simulink model "CANConnectivityInAnAutomotiveApplication4"  (R2024a)
settings: Solver=VariableStepAuto  StartTime=0.0  StopTime=inf  RelTol=1e-3
model workspace (MAT data in the model file):
  k2 = 1e-06
undefined symbols (not defined in the file): canChannel, DiscIntNeverNeededParam
libraries: canmsglib x17, canlib x11, simulink x3
settings Model: Creator=The MathWorks, Inc.  LastModifiedBy=S D
settings SolverCC: AlgebraicLoopSolver=TrustRegion
settings DataIOCC: ReturnWorkspaceOutputs=off
settings DebuggingCC: UnconnectedInputMsg=warning  UnconnectedOutputMsg=warning  UnconnectedLineMsg=warning  ArithmeticOperatorsInVariantConditions=warning
settings ModelReferenceCC: EnableRefExpFcnMdlSchedulingChecks=on
settings SFSimCC: SimUseLocalCustomCode=off  CustomCodeUndefinedFunction=UseInterfaceOnly
settings RTWCC: RTWUseLocalCustomCode=off  GPUComputeCapability=3.5

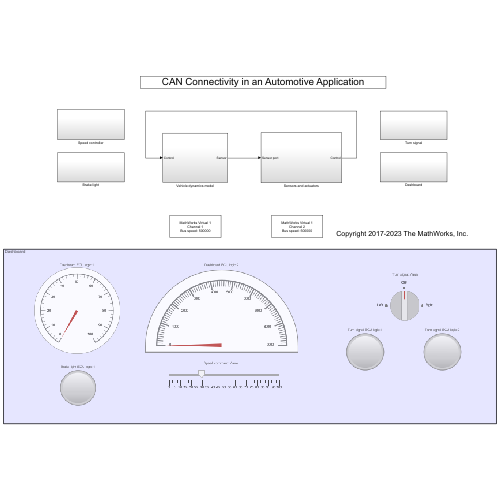
[thumbnail: Simulink's stored preview of the top-level diagram]
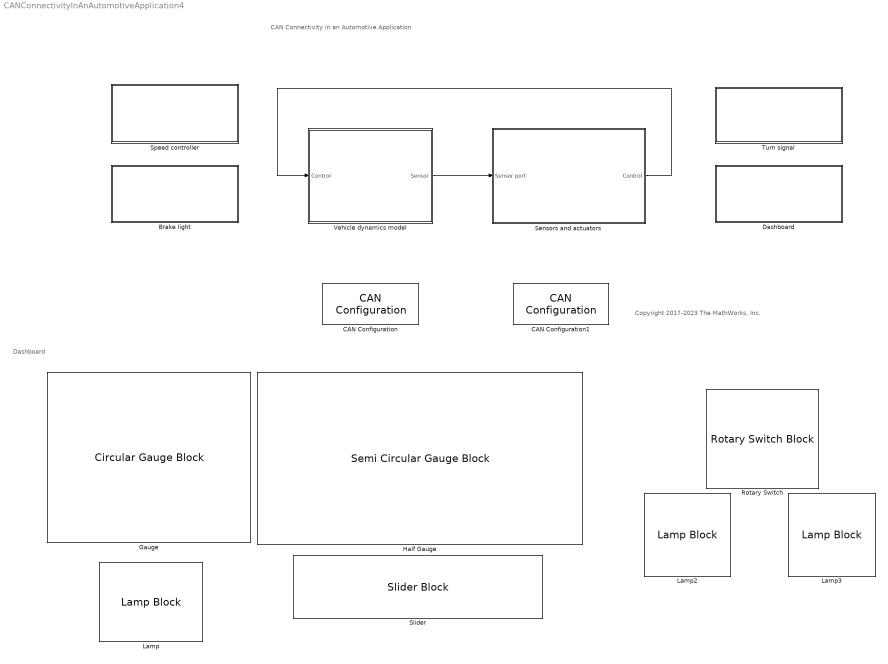
== system CANConnectivityInAnAutomotiveApplication4 ==
  note: Dashboard
  note: CAN Connectivity in an Automotive Application
  note: Copyright 2017-2023 The MathWorks, Inc.
  Brake light : Subsystem
  CAN Configuration : canlib/CAN Configuration  BlockHandle=1838.0012  Device=MathWorks Virtual 1 (Channel 1)  DeviceMenu=MathWorks Virtual 1 (Channel 1)  ObjConstructor=canChannel('MathWorks', 'Virtual 1', 1)  BusSpeed=500000  EnableBitParameters=off  AckMode=Normal
  CAN Configuration1 : canlib/CAN Configuration  BlockHandle=1839.0024  Device=MathWorks Virtual 1 (Channel 2)  DeviceMenu=MathWorks Virtual 1 (Channel 2)  ObjConstructor=canChannel('MathWorks', 'Virtual 1', 2)  BusSpeed=500000  EnableBitParameters=off  AckMode=Normal
  Dashboard : Subsystem
  Gauge : CircularGaugeBlock  TickInterval=10
  Half Gauge : SemiCircularGaugeBlock  ScaleMax=9000  TickInterval=1000
  Lamp : LampBlock
  Lamp2 : LampBlock
  Lamp3 : LampBlock
  Rotary Switch : RotarySwitchBlock
      settings: Values={{'Left', 'Off', 'Right'}, [1 2 3]}
  Sensors and actuators : Subsystem
  Slider : SliderBlock
  Speed controller : Subsystem
  Turn signal : Subsystem
  Vehicle dynamics model : Subsystem
  wires:
  Vehicle dynamics model/1(Sensor) -> Sensors and actuators/1(Sensor port)
  Sensors and actuators/1(Control) -> Vehicle dynamics model/1(Control)

== system CANConnectivityInAnAutomotiveApplication4/Brake light ==
  note: Brake light
  Brake light : Terminator
  Brake light ECU logic : Subsystem  TreatAsAtomicUnit=on
  CAN Receive : canlib/CAN Receive  BlockHandle=1831.002  Device=MathWorks Virtual 1 (Channel 2)  DeviceMenu=MathWorks Virtual 1 (Channel 2)  ObjConstructor=canChannel('MathWorks', 'Virtual 1', 2)  EnableStandardIDsFilter=off  StdIDsCombo=Allow all  StandardIDs=0  EnableExtendedIDsFilter=off  ExtIDsCombo=Allow all  ExtendedIDs=0  SampleTime=0.01  MsgsPerTimestep=all  InternalFilterUpdateStatus=on  BusOutput=on
  wires:
  CAN Receive/1 -> Brake light ECU logic/Trigger
  CAN Receive/2 -> Brake light ECU logic/1(CAN message)
  Brake light ECU logic/1(Brake status) -> Brake light/1

== system CANConnectivityInAnAutomotiveApplication4/Dashboard ==
  note: Dashboard
  CAN Receive : canlib/CAN Receive  BlockHandle=1841.0009  Device=MathWorks Virtual 1 (Channel 2)  DeviceMenu=MathWorks Virtual 1 (Channel 2)  ObjConstructor=canChannel('MathWorks', 'Virtual 1', 2)  EnableStandardIDsFilter=off  StdIDsCombo=Block all  StandardIDs=0  EnableExtendedIDsFilter=off  ExtIDsCombo=Allow all  ExtendedIDs=[50 100]  SampleTime=0.01  MsgsPerTimestep=all  InternalFilterUpdateStatus=on  BusOutput=on
  Dashboard ECU logic : Subsystem  TreatAsAtomicUnit=on
  Speedometer : Terminator
  Tachometer : Terminator
  wires:
  CAN Receive/1 -> Dashboard ECU logic/Trigger
  CAN Receive/2 -> Dashboard ECU logic/1(CAN message)
  Dashboard ECU logic/2(RPM) -> Tachometer/1
  Dashboard ECU logic/1(Speed) -> Speedometer/1

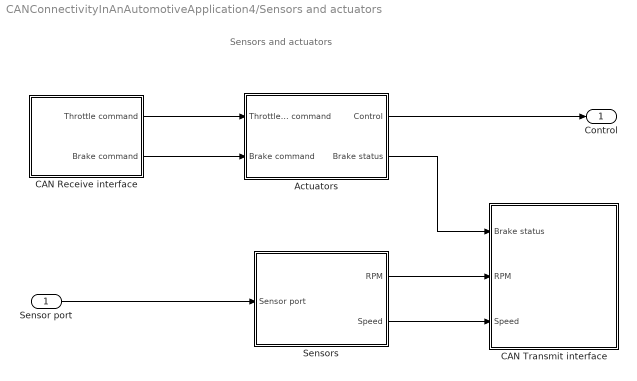
== system CANConnectivityInAnAutomotiveApplication4/Sensors and actuators ==
  note: Sensors and actuators
  Sensor port : Inport
  Actuators : Subsystem
  CAN Receive interface : Subsystem
  CAN Transmit interface : Subsystem
  Sensors : Subsystem
  Control : Outport  VectorParamsAs1DForOutWhenUnconnected=off
  wires:
  Sensor port/1 -> Sensors/1(Sensor port)
  Sensors/1(RPM) -> CAN Transmit interface/2(RPM)
  Sensors/2(Speed) -> CAN Transmit interface/3(Speed)
  Actuators/1(Control) -> Control/1
  Actuators/2(Brake status) -> CAN Transmit interface/1(Brake status)
  CAN Receive interface/1(Throttle command) -> Actuators/1(Throttle command)
  CAN Receive interface/2(Brake command) -> Actuators/2(Brake command)

== system CANConnectivityInAnAutomotiveApplication4/Speed controller ==
  note: Speed controller
  CAN Receive : canlib/CAN Receive  BlockHandle=2493.0005  Device=MathWorks Virtual 1 (Channel 2)  DeviceMenu=MathWorks Virtual 1 (Channel 2)  ObjConstructor=canChannel('MathWorks', 'Virtual 1', 2)  EnableStandardIDsFilter=off  StdIDsCombo=Allow all  StandardIDs=0  EnableExtendedIDsFilter=off  ExtIDsCombo=Allow all  ExtendedIDs=0  SampleTime=0.01  MsgsPerTimestep=all  InternalFilterUpdateStatus=on  BusOutput=on
  Speed controller ECU logic : Subsystem  TreatAsAtomicUnit=on
  wires:
  CAN Receive/1 -> Speed controller ECU logic/Trigger
  CAN Receive/2 -> Speed controller ECU logic/1(CAN message)

== system CANConnectivityInAnAutomotiveApplication4/Turn signal ==
  note: Turn signal
  CAN Receive : canlib/CAN Receive  BlockHandle=2632.0002  Device=MathWorks Virtual 1 (Channel 2)  DeviceMenu=MathWorks Virtual 1 (Channel 2)  ObjConstructor=canChannel('MathWorks', 'Virtual 1', 2)  EnableStandardIDsFilter=off  StdIDsCombo=Block all  StandardIDs=0  EnableExtendedIDsFilter=off  ExtIDsCombo=Allow all  ExtendedIDs=600  SampleTime=0.01  MsgsPerTimestep=all  InternalFilterUpdateStatus=on  BusOutput=on
  Left turn signal : Terminator
  Right turn signal : Terminator
  Turn signal ECU logic : Subsystem  TreatAsAtomicUnit=on
  wires:
  CAN Receive/1 -> Turn signal ECU logic/Trigger
  CAN Receive/2 -> Turn signal ECU logic/1(CAN message)
  Turn signal ECU logic/1(Left turn signal interface) -> Left turn signal/1
  Turn signal ECU logic/2(Right turn signal interface) -> Right turn signal/1

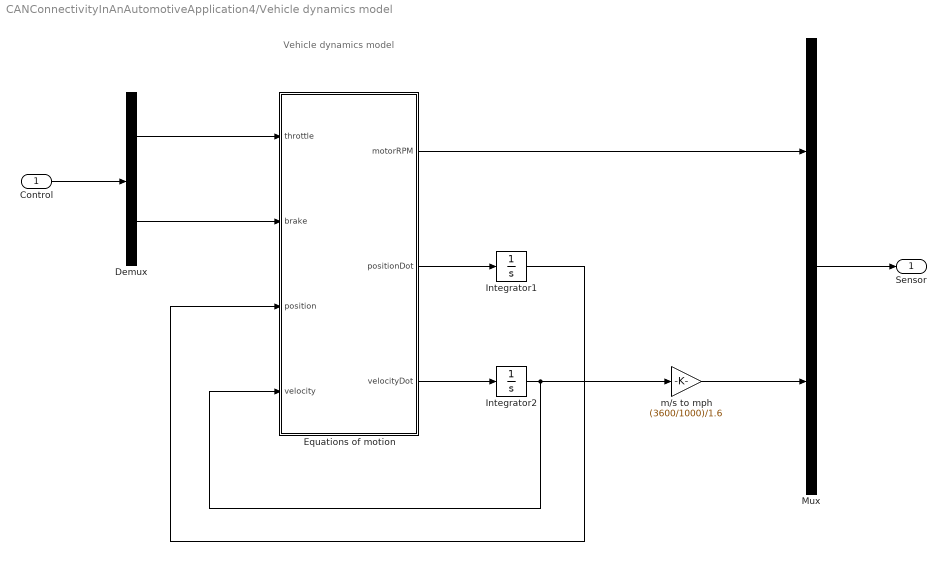
== system CANConnectivityInAnAutomotiveApplication4/Vehicle dynamics model ==
  note: Vehicle dynamics model
  Control : Inport
  Demux : Demux  Outputs=2
  Equations of motion : MATLAB Function  TreatAsAtomicUnit=on
  Integrator1 : Integrator
  Integrator2 : Integrator
  Mux : Mux  Inputs=2
  m/s to mph : Gain  Gain=(3600/1000)/1.6
  Sensor : Outport  VectorParamsAs1DForOutWhenUnconnected=off
  wires:
  Demux/1 -> Equations of motion/1(throttle)
  Equations of motion/2(positionDot) -> Integrator1/1
  Equations of motion/3(velocityDot) -> Integrator2/1
  Integrator2/1 -> m/s to mph/1, Equations of motion/4(velocity)
  Integrator1/1 -> Equations of motion/3(position)
  Demux/2 -> Equations of motion/2(brake)
  m/s to mph/1 -> Mux/2
  Equations of motion/1(motorRPM) -> Mux/1
  Control/1 -> Demux/1
  Mux/1 -> Sensor/1

== system CANConnectivityInAnAutomotiveApplication4/Brake light/Brake light ECU logic ==
  note: Brake light ECU logic
  CAN message : Inport
  function : TriggerPort  TriggerType=function-call  VariantControl=Variant
  CAN Unpack : canmsglib/CAN Unpack  CANdbFile=canConnectivityForVehicle.dbc  MsgList=BrakeStatusMessage  MsgName=BrakeStatusMessage  MsgIDType=Extended (29-bit identifier)  MsgIdentifier=1280  MsgLength=1  SignalInfo={'BrakeStatus','0','1','LE','unsigned','Standard','0','1','0','0','1'}  IDPort=off  TimestampPort=off  ErrorPort=off  RemotePort=off  LengthPort=off  StatusPort=off  ApplyMinMax=off
      settings: DataFormat=CANdb specified signals
  Brake status : Outport  VectorParamsAs1DForOutWhenUnconnected=off
  wires:
  CAN message/1 -> CAN Unpack/1
  CAN Unpack/1 -> Brake status/1

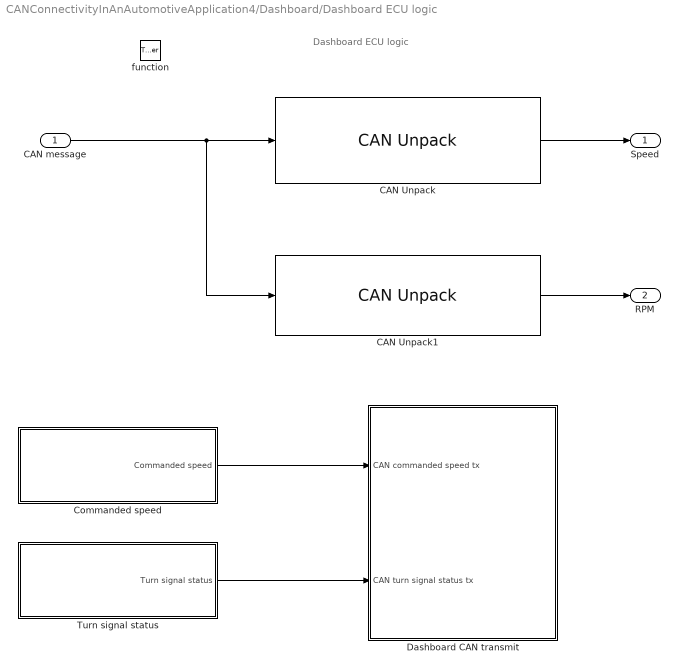
== system CANConnectivityInAnAutomotiveApplication4/Dashboard/Dashboard ECU logic ==
  note: Dashboard ECU logic
  CAN message : Inport
  function : TriggerPort  TriggerType=function-call  VariantControl=Variant
  CAN Unpack : canmsglib/CAN Unpack  CANdbFile=canConnectivityForVehicle.dbc  MsgList=SpeedMessage  MsgName=SpeedMessage  MsgIDType=Extended (29-bit identifier)  MsgIdentifier=256  MsgLength=8  SignalInfo={'Speed','0','64','LE','double','Standard','0','1','0','0','100'}  IDPort=off  TimestampPort=off  ErrorPort=off  RemotePort=off  LengthPort=off  StatusPort=off  ApplyMinMax=off
      settings: DataFormat=CANdb specified signals
  CAN Unpack1 : canmsglib/CAN Unpack  CANdbFile=canConnectivityForVehicle.dbc  MsgList=RPMMessage  MsgName=RPMMessage  MsgIDType=Extended (29-bit identifier)  MsgIdentifier=2048  MsgLength=8  SignalInfo={'RPM','0','64','LE','double','Standard','0','1','0','0','10000'}  IDPort=off  TimestampPort=off  ErrorPort=off  RemotePort=off  LengthPort=off  StatusPort=off  ApplyMinMax=off
      settings: DataFormat=CANdb specified signals
  Commanded speed : Subsystem
  Dashboard CAN transmit : Subsystem
  Turn signal status : Subsystem
  Speed : Outport  VectorParamsAs1DForOutWhenUnconnected=off
  RPM : Outport  Port=2  VectorParamsAs1DForOutWhenUnconnected=off
  wires:
  CAN message/1 -> CAN Unpack1/1, CAN Unpack/1
  Turn signal status/1(Turn signal status) -> Dashboard CAN transmit/2(CAN turn signal status tx)
  Commanded speed/1(Commanded speed) -> Dashboard CAN transmit/1(CAN commanded speed tx)
  CAN Unpack/1 -> Speed/1
  CAN Unpack1/1 -> RPM/1

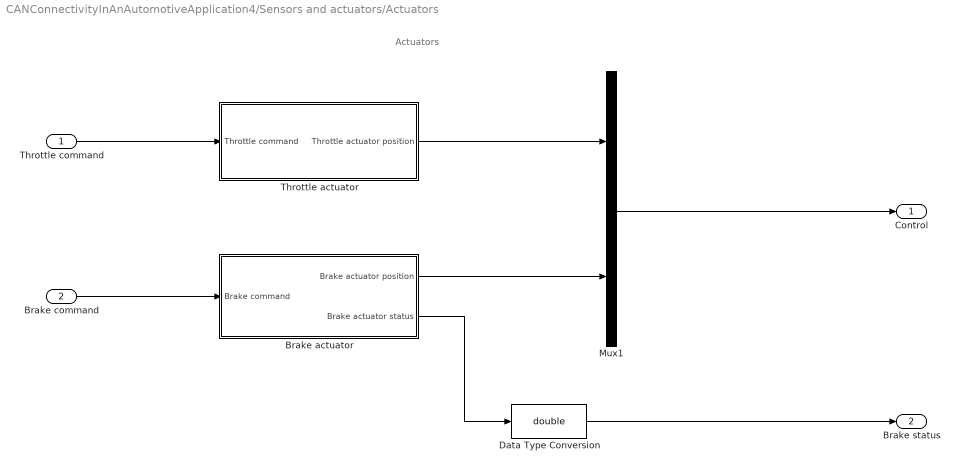
== system CANConnectivityInAnAutomotiveApplication4/Sensors and actuators/Actuators ==
  note: Actuators
  Throttle command : Inport
  Brake command : Inport  Port=2
  Brake actuator : Subsystem
  Data Type Conversion : DataTypeConversion  OutDataTypeStr=double  SaturateOnIntegerOverflow=off  RndMeth=Floor
  Mux1 : Mux  Inputs=2
  Throttle actuator : Subsystem
  Control : Outport  VectorParamsAs1DForOutWhenUnconnected=off
  Brake status : Outport  Port=2  VectorParamsAs1DForOutWhenUnconnected=off
  wires:
  Brake actuator/1(Brake actuator position) -> Mux1/2
  Throttle actuator/1(Throttle actuator position) -> Mux1/1
  Brake command/1 -> Brake actuator/1(Brake command)
  Throttle command/1 -> Throttle actuator/1(Throttle command)
  Data Type Conversion/1 -> Brake status/1
  Brake actuator/2(Brake actuator status) -> Data Type Conversion/1
  Mux1/1 -> Control/1

== system CANConnectivityInAnAutomotiveApplication4/Sensors and actuators/CAN Receive interface ==
  note: CAN Receive interface
  CAN Receive : canlib/CAN Receive  BlockHandle=2311.0005  Device=MathWorks Virtual 1 (Channel 1)  DeviceMenu=MathWorks Virtual 1 (Channel 1)  ObjConstructor=canChannel('MathWorks', 'Virtual 1', 1)  EnableStandardIDsFilter=off  StdIDsCombo=Allow all  StandardIDs=0  EnableExtendedIDsFilter=off  ExtIDsCombo=Allow all  ExtendedIDs=0  SampleTime=0.01  MsgsPerTimestep=all  InternalFilterUpdateStatus=off  BusOutput=on
  Extract message : Subsystem  TreatAsAtomicUnit=on
  Throttle command : Outport  VectorParamsAs1DForOutWhenUnconnected=off
  Brake command : Outport  Port=2  VectorParamsAs1DForOutWhenUnconnected=off
  wires:
  CAN Receive/1 -> Extract message/Trigger
  CAN Receive/2 -> Extract message/1(In1)
  Extract message/1(Throttle command) -> Throttle command/1
  Extract message/2(Brake actuator position) -> Brake command/1

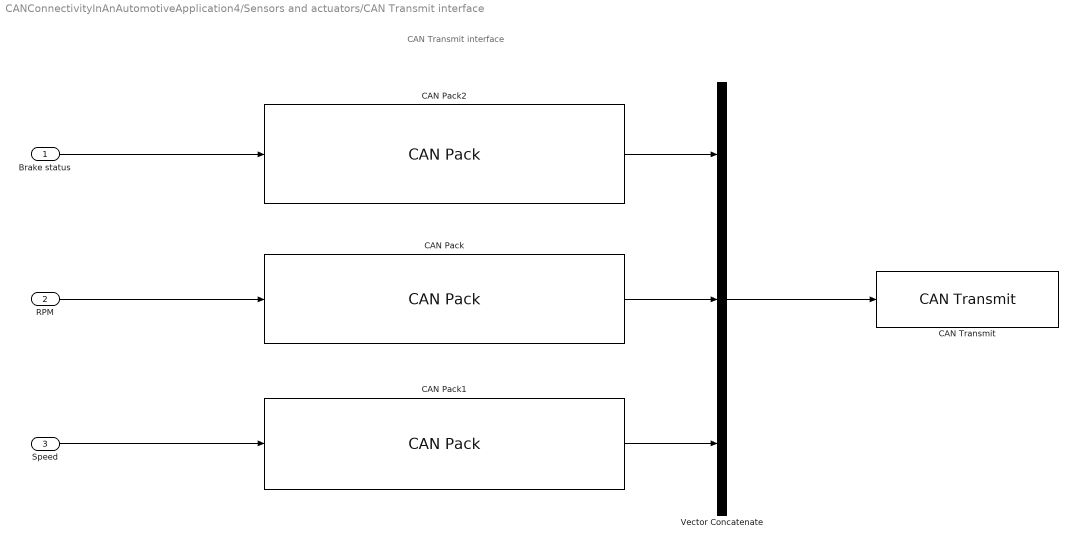
== system CANConnectivityInAnAutomotiveApplication4/Sensors and actuators/CAN Transmit interface ==
  note: CAN Transmit interface
  Brake status : Inport
  RPM : Inport  Port=2
  Speed : Inport  Port=3
  CAN Pack : canmsglib/CAN Pack  CANdbFile=canConnectivityForVehicle.dbc  MsgList=RPMMessage  MsgName=RPMMessage  MsgIDType=Extended (29-bit identifier)  MsgIdentifier=2048  MsgLength=8  Remote=off  ApplyMinMax=off  BusOutput=on  SignalInfo={'RPM','0','64','LE','double','Standard','0','1','0','0','10000'}
      settings: DataFormat=CANdb specified signals
  CAN Pack1 : canmsglib/CAN Pack  CANdbFile=canConnectivityForVehicle.dbc  MsgList=SpeedMessage  MsgName=SpeedMessage  MsgIDType=Extended (29-bit identifier)  MsgIdentifier=256  MsgLength=8  Remote=off  ApplyMinMax=off  BusOutput=on  SignalInfo={'Speed','0','64','LE','double','Standard','0','1','0','0','100'}
      settings: DataFormat=CANdb specified signals
  CAN Pack2 : canmsglib/CAN Pack  CANdbFile=canConnectivityForVehicle.dbc  MsgList=BrakeStatusMessage  MsgName=BrakeStatusMessage  MsgIDType=Extended (29-bit identifier)  MsgIdentifier=1280  MsgLength=1  Remote=off  ApplyMinMax=off  BusOutput=on  SignalInfo={'BrakeStatus','0','1','LE','unsigned','Standard','0','1','0','0','1'}
      settings: DataFormat=CANdb specified signals
  CAN Transmit : canlib/CAN Transmit  BlockHandle=2420.0005  Device=MathWorks Virtual 1 (Channel 1)  DeviceMenu=MathWorks Virtual 1 (Channel 1)  ObjConstructor=canChannel('MathWorks', 'Virtual 1', 1)  EnableEventTransmit=off  EnablePeriodicTransmit=off  MessagePeriod=1.000
  Vector Concatenate : Concatenate  NumInputs=3
  wires:
  Speed/1 -> CAN Pack1/1
  Brake status/1 -> CAN Pack2/1
  CAN Pack1/1 -> Vector Concatenate/3
  Vector Concatenate/1 -> CAN Transmit/1
  CAN Pack/1 -> Vector Concatenate/2
  CAN Pack2/1 -> Vector Concatenate/1
  RPM/1 -> CAN Pack/1

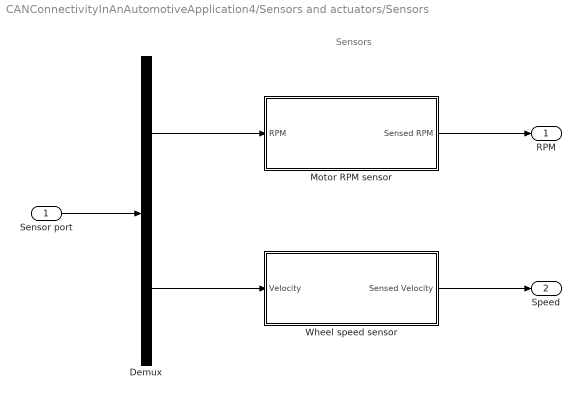
== system CANConnectivityInAnAutomotiveApplication4/Sensors and actuators/Sensors ==
  note: Sensors
  Sensor port : Inport
  Demux : Demux  Outputs=2
  Motor RPM sensor : Subsystem
  Wheel speed sensor : Subsystem
  RPM : Outport  VectorParamsAs1DForOutWhenUnconnected=off
  Speed : Outport  Port=2  VectorParamsAs1DForOutWhenUnconnected=off
  wires:
  Motor RPM sensor/1(Sensed RPM) -> RPM/1
  Wheel speed sensor/1(Sensed Velocity) -> Speed/1
  Demux/1 -> Motor RPM sensor/1(RPM)
  Demux/2 -> Wheel speed sensor/1(Velocity)
  Sensor port/1 -> Demux/1

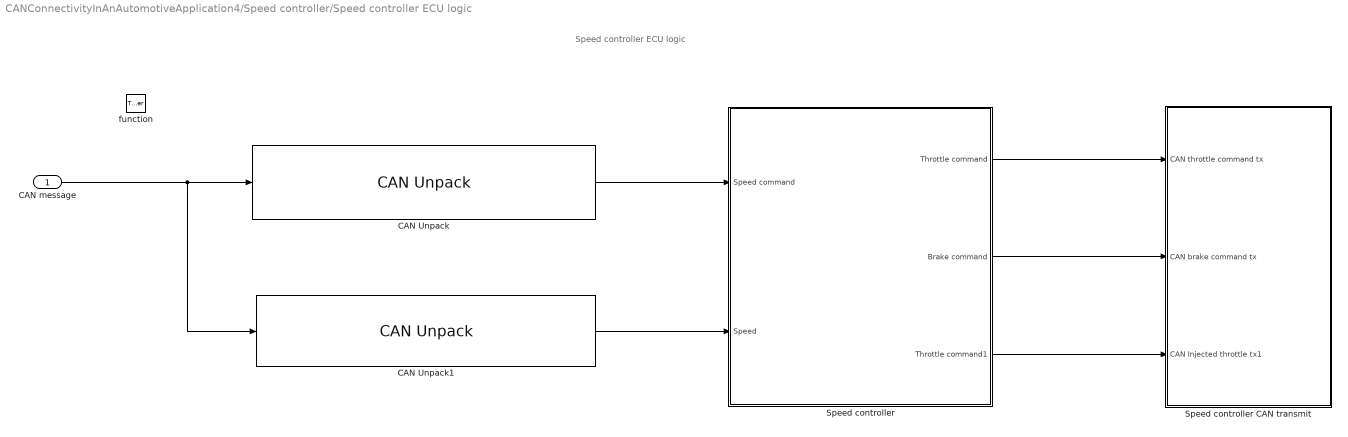
== system CANConnectivityInAnAutomotiveApplication4/Speed controller/Speed controller ECU logic ==
  note: Speed controller ECU logic
  CAN message : Inport
  function : TriggerPort  TriggerType=function-call  VariantControl=Variant
  CAN Unpack : canmsglib/CAN Unpack  CANdbFile=canConnectivityForVehicle.dbc  MsgList=SpeedCommandMessage  MsgName=SpeedCommandMessage  MsgIDType=Extended (29-bit identifier)  MsgIdentifier=1024  MsgLength=8  SignalInfo={'SpeedCommand','0','64','LE','double','Standard','0','1','0','0','100'}  IDPort=off  TimestampPort=off  ErrorPort=off  RemotePort=off  LengthPort=off  StatusPort=off  ApplyMinMax=off
      settings: DataFormat=CANdb specified signals
  CAN Unpack1 : canmsglib/CAN Unpack  CANdbFile=canConnectivityForVehicle.dbc  MsgList=SpeedMessage  MsgName=SpeedMessage  MsgIDType=Extended (29-bit identifier)  MsgIdentifier=256  MsgLength=8  SignalInfo={'Speed','0','64','LE','double','Standard','0','1','0','0','100'}  IDPort=off  TimestampPort=off  ErrorPort=off  RemotePort=off  LengthPort=off  StatusPort=off  ApplyMinMax=off
      settings: DataFormat=CANdb specified signals
  Speed controller : Subsystem
  Speed controller CAN transmit : Subsystem
  wires:
  CAN message/1 -> CAN Unpack1/1, CAN Unpack/1
  Speed controller/1(Throttle command) -> Speed controller CAN transmit/1(CAN throttle command tx)
  Speed controller/2(Brake command) -> Speed controller CAN transmit/2(CAN brake command tx)
  CAN Unpack/1 -> Speed controller/1(Speed command)
  CAN Unpack1/1 -> Speed controller/2(Speed)
  Speed controller/3(Throttle command1) -> Speed controller CAN transmit/3(CAN Injected throttle tx1)

== system CANConnectivityInAnAutomotiveApplication4/Turn signal/Turn signal ECU logic ==
  note: Turn signal ECU logic
  CAN message : Inport
  function : TriggerPort  TriggerType=function-call  VariantControl=Variant
  CAN Unpack : canmsglib/CAN Unpack  CANdbFile=canConnectivityForVehicle.dbc  MsgList=TurnSignalStatusMessage  MsgName=TurnSignalStatusMessage  MsgIDType=Extended (29-bit identifier)  MsgIdentifier=1536  MsgLength=1  SignalInfo={'TurnSignalStatus','0','3','LE','unsigned','Standard','0','1','0','1','3'}  IDPort=off  TimestampPort=off  ErrorPort=off  RemotePort=off  LengthPort=off  StatusPort=off  ApplyMinMax=off
      settings: DataFormat=CANdb specified signals
  Turn signal logic : Subsystem
  Left turn signal interface : Outport  VectorParamsAs1DForOutWhenUnconnected=off
  Right turn signal interface : Outport  Port=2  VectorParamsAs1DForOutWhenUnconnected=off
  wires:
  CAN message/1 -> CAN Unpack/1
  CAN Unpack/1 -> Turn signal logic/1(Turn signal status)
  Turn signal logic/1(Left turn signal interface) -> Left turn signal interface/1
  Turn signal logic/2(Right turn signal interface) -> Right turn signal interface/1

== system CANConnectivityInAnAutomotiveApplication4/Dashboard/Dashboard ECU logic/Commanded speed ==
  note: Commanded speed
  Speed command : Constant  Value=42.53198205682007  OutDataTypeStr=double  SampleTime=Inf
  Zero-Order Hold : ZeroOrderHold  SampleTime=-1
  Commanded speed : Outport  VectorParamsAs1DForOutWhenUnconnected=off
  wires:
  Speed command/1 -> Zero-Order Hold/1
  Zero-Order Hold/1 -> Commanded speed/1

== system CANConnectivityInAnAutomotiveApplication4/Dashboard/Dashboard ECU logic/Dashboard CAN transmit ==
  note: Dashboard CAN transmit
  CAN commanded speed tx : Inport
  CAN turn signal status tx : Inport  Port=2
  CAN Pack : canmsglib/CAN Pack  CANdbFile=canConnectivityForVehicle.dbc  MsgList=TurnSignalStatusMessage  MsgName=TurnSignalStatusMessage  MsgIDType=Extended (29-bit identifier)  MsgIdentifier=1536  MsgLength=1  Remote=off  ApplyMinMax=off  BusOutput=on  SignalInfo={'TurnSignalStatus','0','3','LE','unsigned','Standard','0','1','0','1','3'}
      settings: DataFormat=CANdb specified signals
  CAN Pack1 : canmsglib/CAN Pack  CANdbFile=canConnectivityForVehicle.dbc  MsgList=SpeedCommandMessage  MsgName=SpeedCommandMessage  MsgIDType=Extended (29-bit identifier)  MsgIdentifier=1024  MsgLength=8  Remote=off  ApplyMinMax=off  BusOutput=on  SignalInfo={'SpeedCommand','0','64','LE','double','Standard','0','1','0','0','100'}
      settings: DataFormat=CANdb specified signals
  CAN Transmit : canlib/CAN Transmit  BlockHandle=1905.0026  Device=MathWorks Virtual 1 (Channel 1)  DeviceMenu=MathWorks Virtual 1 (Channel 1)  ObjConstructor=canChannel('MathWorks', 'Virtual 1', 1)  EnableEventTransmit=off  EnablePeriodicTransmit=on  MessagePeriod=0.01
  CAN Transmit1 : canlib/CAN Transmit  BlockHandle=1907.0023  Device=MathWorks Virtual 1 (Channel 1)  DeviceMenu=MathWorks Virtual 1 (Channel 1)  ObjConstructor=canChannel('MathWorks', 'Virtual 1', 1)  EnableEventTransmit=off  EnablePeriodicTransmit=on  MessagePeriod=0.01
  wires:
  CAN commanded speed tx/1 -> CAN Pack1/1
  CAN Pack/1 -> CAN Transmit/1
  CAN turn signal status tx/1 -> CAN Pack/1
  CAN Pack1/1 -> CAN Transmit1/1

== system CANConnectivityInAnAutomotiveApplication4/Dashboard/Dashboard ECU logic/Turn signal status ==
  note: Turn signal status
  Turn signal : Constant  Value=2  OutDataTypeStr=double
  Zero-Order Hold : ZeroOrderHold  SampleTime=-1
  Turn signal status : Outport  VectorParamsAs1DForOutWhenUnconnected=off
  wires:
  Turn signal/1 -> Zero-Order Hold/1
  Zero-Order Hold/1 -> Turn signal status/1

== system CANConnectivityInAnAutomotiveApplication4/Sensors and actuators/Actuators/Brake actuator ==
  note: Brake actuator
  Brake command : Inport
  Brake actuator : TransferFcn  Denominator=[0.1 1]
  Brake status sensor : Subsystem
  Brake actuator position : Outport  VectorParamsAs1DForOutWhenUnconnected=off
  Brake actuator status : Outport  Port=2  VectorParamsAs1DForOutWhenUnconnected=off
  wires:
  Brake status sensor/1(Brake status) -> Brake actuator status/1
  Brake command/1 -> Brake actuator/1
  Brake actuator/1 -> Brake actuator position/1, Brake status sensor/1(Brake actuator position)

== system CANConnectivityInAnAutomotiveApplication4/Sensors and actuators/Actuators/Throttle actuator ==
  note: Throttle actuator
  Throttle command : Inport
  Throttle actuator : TransferFcn  Denominator=[0.1 1]
  Throttle actuator position : Outport  VectorParamsAs1DForOutWhenUnconnected=off
  wires:
  Throttle command/1 -> Throttle actuator/1
  Throttle actuator/1 -> Throttle actuator position/1

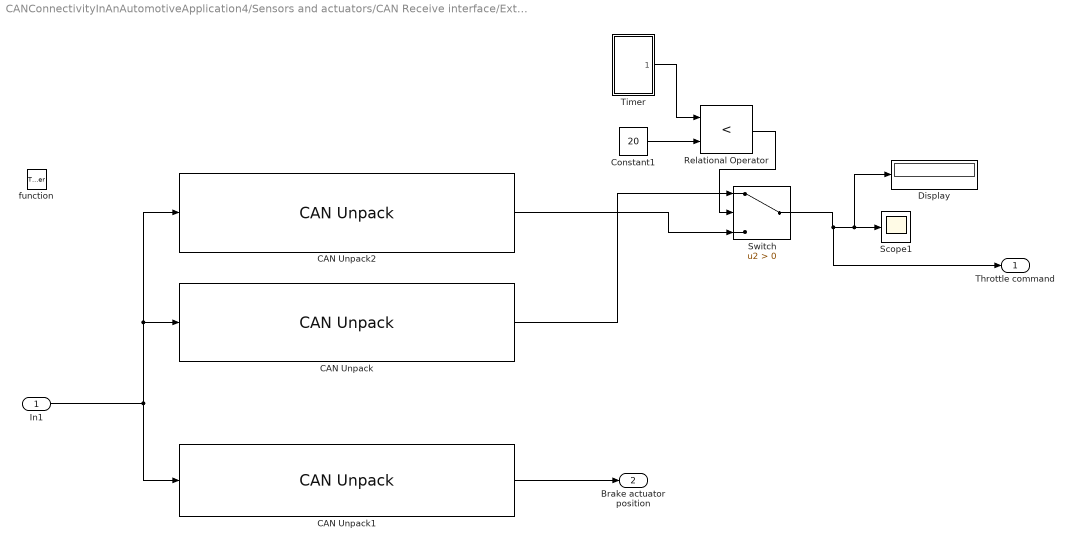
== system CANConnectivityInAnAutomotiveApplication4/Sensors and actuators/CAN Receive interface/Extract message ==
  In1 : Inport
  function : TriggerPort  TriggerType=function-call  VariantControl=Variant
  CAN Unpack : canmsglib/CAN Unpack  CANdbFile=canConnectivityForVehicle.dbc  MsgList=ThrottleCommandMessage  MsgName=ThrottleCommandMessage  MsgIDType=Extended (29-bit identifier)  MsgIdentifier=96  MsgLength=8  SignalInfo={'ThrottleCommand','0','64','LE','double','Standard','0','1','0','0','1'}  IDPort=off  TimestampPort=off  ErrorPort=off  RemotePort=off  LengthPort=off  StatusPort=off  ApplyMinMax=off
      settings: DataFormat=CANdb specified signals
  CAN Unpack1 : canmsglib/CAN Unpack  CANdbFile=canConnectivityForVehicle.dbc  MsgList=BrakeCommandMessage  MsgName=BrakeCommandMessage  MsgIDType=Extended (29-bit identifier)  MsgIdentifier=81  MsgLength=8  SignalInfo={'BrakeCommand','0','64','LE','double','Standard','0','1','0','0','1'}  IDPort=off  TimestampPort=off  ErrorPort=off  RemotePort=off  LengthPort=off  StatusPort=off  ApplyMinMax=off
      settings: DataFormat=CANdb specified signals
  CAN Unpack2 : canmsglib/CAN Unpack  CANdbFile=canConnectivityForVehicle.dbc  MsgList=InjectedThrottleMessage  MsgName=InjectedThrottleMessage  MsgIDType=Extended (29-bit identifier)  MsgIdentifier=95  MsgLength=8  SignalInfo={'InjectedThrottle','0','64','LE','double','Standard','0','0.5','0','0','0.5'}  IDPort=off  TimestampPort=off  ErrorPort=off  RemotePort=off  LengthPort=off  StatusPort=off  ApplyMinMax=off
      settings: DataFormat=CANdb specified signals
  Constant1 : Constant  Value=20
  Display : Display
  Relational Operator : RelationalOperator  Operator=<  OutDataTypeStr=boolean  RndMeth=Simplest  InputSameDT=off
  Scope1 : Scope
  Switch : Switch  Criteria=u2 > Threshold  SaturateOnIntegerOverflow=off  InputSameDT=off
  Timer : Subsystem
  Throttle command : Outport  VectorParamsAs1DForOutWhenUnconnected=off
  Brake actuator position : Outport  Port=2  VectorParamsAs1DForOutWhenUnconnected=off
  wires:
  In1/1 -> CAN Unpack1/1, CAN Unpack2/1, CAN Unpack/1
  CAN Unpack1/1 -> Brake actuator position/1
  Relational Operator/1 -> Switch/2
  Timer/1(Outport) -> Relational Operator/1
  Constant1/1 -> Relational Operator/2
  Switch/1 -> Throttle command/1, Display/1, Scope1/1
  CAN Unpack/1 -> Switch/1
  CAN Unpack2/1 -> Switch/3

== system CANConnectivityInAnAutomotiveApplication4/Sensors and actuators/Sensors/Motor RPM sensor ==
  note: Motor RPM sensor
  RPM : Inport
  Zero-Order Hold : ZeroOrderHold  SampleTime=.01
  Sensed RPM : Outport  VectorParamsAs1DForOutWhenUnconnected=off
  wires:
  Zero-Order Hold/1 -> Sensed RPM/1
  RPM/1 -> Zero-Order Hold/1

== system CANConnectivityInAnAutomotiveApplication4/Sensors and actuators/Sensors/Wheel speed sensor ==
  note: Wheel speed sensor
  Velocity : Inport
  Zero-Order Hold : ZeroOrderHold  SampleTime=.01
  Sensed Velocity : Outport  VectorParamsAs1DForOutWhenUnconnected=off
  wires:
  Zero-Order Hold/1 -> Sensed Velocity/1
  Velocity/1 -> Zero-Order Hold/1

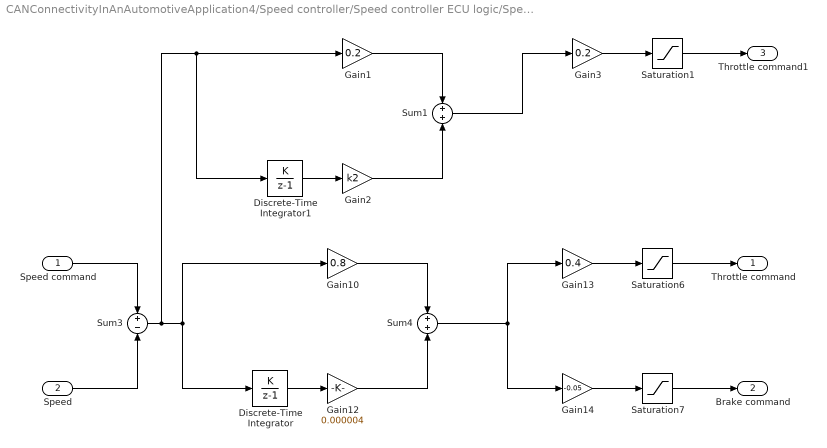
== system CANConnectivityInAnAutomotiveApplication4/Speed controller/Speed controller ECU logic/Speed controller ==
  Speed command : Inport
  Speed : Inport  Port=2
  Discrete-Time Integrator : DiscreteIntegrator  IntegratorMethod=Accumulation: Forward Euler  SampleTime=-1  ICPrevOutput=DiscIntNeverNeededParam  ICPrevScaledInput=DiscIntNeverNeededParam
  Discrete-Time Integrator1 : DiscreteIntegrator  IntegratorMethod=Accumulation: Forward Euler  SampleTime=-1  ICPrevOutput=DiscIntNeverNeededParam  ICPrevScaledInput=DiscIntNeverNeededParam
  Gain1 : Gain  Gain=0.2
  Gain10 : Gain  Gain=0.8
  Gain12 : Gain  Gain=0.000004
  Gain13 : Gain  Gain=0.4
  Gain14 : Gain  Gain=-0.05
  Gain2 : Gain  Gain=k2
  Gain3 : Gain  Gain=0.2
  Saturation1 : Saturate  UpperLimit=1  LowerLimit=0
  Saturation6 : Saturate  UpperLimit=1  LowerLimit=0
  Saturation7 : Saturate  UpperLimit=1  LowerLimit=0
  Sum1 : Sum  Inputs=+|+
  Sum3 : Sum  Inputs=+|-
  Sum4 : Sum  Inputs=+|+
  Throttle command : Outport  VectorParamsAs1DForOutWhenUnconnected=off
  Brake command : Outport  Port=2  VectorParamsAs1DForOutWhenUnconnected=off
  Throttle command1 : Outport  Port=3  VectorParamsAs1DForOutWhenUnconnected=off
  wires:
  Saturation7/1 -> Brake command/1
  Saturation6/1 -> Throttle command/1
  Speed command/1 -> Sum3/1
  Speed/1 -> Sum3/2
  Sum3/1 -> Discrete-Time Integrator1/1, Gain1/1, Discrete-Time Integrator/1, Gain10/1
  Discrete-Time Integrator/1 -> Gain12/1
  Gain10/1 -> Sum4/1
  Sum4/1 -> Gain14/1, Gain13/1
  Gain14/1 -> Saturation7/1
  Gain13/1 -> Saturation6/1
  Gain12/1 -> Sum4/2
  Gain3/1 -> Saturation1/1
  Saturation1/1 -> Throttle command1/1
  Gain2/1 -> Sum1/2
  Gain1/1 -> Sum1/1
  Discrete-Time Integrator1/1 -> Gain2/1
  Sum1/1 -> Gain3/1

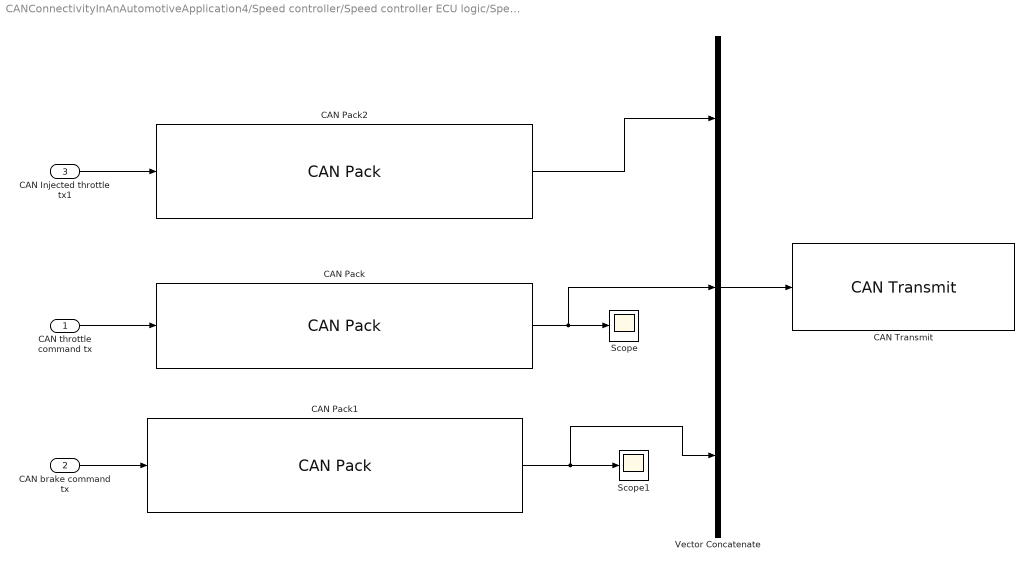
== system CANConnectivityInAnAutomotiveApplication4/Speed controller/Speed controller ECU logic/Speed controller CAN transmit ==
  CAN throttle command tx : Inport
  CAN brake command tx : Inport  Port=2
  CAN Injected throttle tx1 : Inport  Port=3
  CAN Pack : canmsglib/CAN Pack  CANdbFile=canConnectivityForVehicle.dbc  MsgList=ThrottleCommandMessage  MsgName=ThrottleCommandMessage  MsgIDType=Extended (29-bit identifier)  MsgIdentifier=96  MsgLength=8  Remote=off  ApplyMinMax=off  BusOutput=on  SignalInfo={'ThrottleCommand','0','64','LE','double','Standard','0','1','0','0','1'}
      settings: DataFormat=CANdb specified signals
  CAN Pack1 : canmsglib/CAN Pack  CANdbFile=canConnectivityForVehicle.dbc  MsgList=BrakeCommandMessage  MsgName=BrakeCommandMessage  MsgIDType=Extended (29-bit identifier)  MsgIdentifier=81  MsgLength=8  Remote=off  ApplyMinMax=off  BusOutput=on  SignalInfo={'BrakeCommand','0','64','LE','double','Standard','0','1','0','0','1'}
      settings: DataFormat=CANdb specified signals
  CAN Pack2 : canmsglib/CAN Pack  CANdbFile=canConnectivityForVehicle.dbc  MsgList=InjectedThrottleMessage  MsgName=InjectedThrottleMessage  MsgIDType=Extended (29-bit identifier)  MsgIdentifier=95  MsgLength=8  Remote=off  ApplyMinMax=off  BusOutput=on  SignalInfo={'InjectedThrottle','0','64','LE','double','Standard','0','0.5','0','0','0.5'}
      settings: DataFormat=CANdb specified signals
  CAN Transmit : canlib/CAN Transmit  BlockHandle=2597.0002  Device=MathWorks Virtual 1 (Channel 1)  DeviceMenu=MathWorks Virtual 1 (Channel 1)  ObjConstructor=canChannel('MathWorks', 'Virtual 1', 1)  EnableEventTransmit=off  EnablePeriodicTransmit=on  MessagePeriod=0.01
  Scope : Scope
  Scope1 : Scope
  Vector Concatenate : Concatenate  NumInputs=3
  wires:
  CAN Pack/1 -> Vector Concatenate/2, Scope/1
  CAN throttle command tx/1 -> CAN Pack/1
  CAN brake command tx/1 -> CAN Pack1/1
  Vector Concatenate/1 -> CAN Transmit/1
  CAN Pack1/1 -> Vector Concatenate/3, Scope1/1
  CAN Injected throttle tx1/1 -> CAN Pack2/1
  CAN Pack2/1 -> Vector Concatenate/1

== system CANConnectivityInAnAutomotiveApplication4/Turn signal/Turn signal ECU logic/Turn signal logic ==
  note: Turn signal logic
  Turn signal status : Inport
  Compare To Constant1 : simulink/Logic and Bit Operations/Compare To Constant  relop===  const=1  OutDataTypeStr=boolean
  Compare To Constant2 : simulink/Logic and Bit Operations/Compare To Constant  relop===  const=3  OutDataTypeStr=boolean
  Left turn signal interface : Outport  VectorParamsAs1DForOutWhenUnconnected=off
  Right turn signal interface : Outport  Port=2  VectorParamsAs1DForOutWhenUnconnected=off
  wires:
  Turn signal status/1 -> Compare To Constant2/1, Compare To Constant1/1
  Compare To Constant2/1 -> Right turn signal interface/1
  Compare To Constant1/1 -> Left turn signal interface/1

== system CANConnectivityInAnAutomotiveApplication4/Sensors and actuators/Actuators/Brake actuator/Brake status sensor ==
  note: Brake status sensor
  Brake actuator position : Inport
  Compare To Constant : simulink/Logic and Bit Operations/Compare To Constant  relop=>  const=0.01  OutDataTypeStr=boolean
  Zero-Order Hold : ZeroOrderHold  SampleTime=0.01
  Brake status : Outport  VectorParamsAs1DForOutWhenUnconnected=off
  wires:
  Zero-Order Hold/1 -> Brake status/1
  Brake actuator position/1 -> Compare To Constant/1
  Compare To Constant/1 -> Zero-Order Hold/1

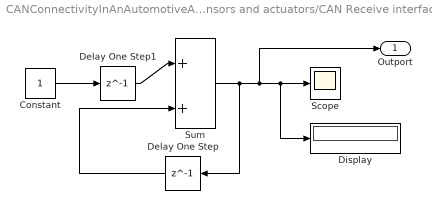
== system CANConnectivityInAnAutomotiveApplication4/Sensors and actuators/CAN Receive interface/Extract message/Timer ==
  Constant : Constant
  Delay One Step : Delay  DelayLength=1
  Delay One Step1 : Delay  DelayLength=1
  Display : Display
  Scope : Scope
  Sum : Sum  Inputs=|++
  Outport : Outport
  wires:
  Sum/1 -> Delay One Step/1, Outport/1, Display/1, Scope/1
  Delay One Step1/1 -> Sum/1
  Constant/1 -> Delay One Step1/1
  Delay One Step/1 -> Sum/2

== matlab function CANConnectivityInAnAutomotiveApplication4/Vehicle dynamics model/Equations of motion ==
  data: throttle input; brake input; position input; motorRPM output; positionDot output; velocity input; velocityDot output
function [motorRPM, positionDot, velocityDot] = car(throttle, brake, position, velocity) %#ok<INUSL>
% This function defines the equations of motion of the vehicle. The vehicle
% is powered by an electric motor with a gearbox. The gear ratio from the
% motor to the wheels is 6:1.

% Radius of wheel
wheelRadius = 0.3;

% Define the mass properties 
wheelMass = 10;
chassisMass = 1300;
wheelMomentOfInertia = 0.5*wheelMass*wheelRadius*wheelRadius;
mass = (4*wheelMass) + chassisMass + (4 * wheelMomentOfInertia/(wheelRadius^2));

% Compute the motor RPM fromt he wheel speed assuming that the wheels don't
% slip.
motorRPM = (velocity/wheelRadius)*(60/(2*pi))*6;

% Compute the upper bound of the motor torque for the current RPM.
motorTorqueUpperBound = 300*exp(-(0.0001*motorRPM));

% Compute the forces acting on the vehicle.
dragForce = 0.5*1.225*(velocity^2)*2;
totalFrictionForce = 0.4*velocity;
motorForce = throttle*motorTorqueUpperBound*6/wheelRadius;
brakeForce = brake*sign(velocity)*1600/wheelRadius;
force = motorForce - dragForce - totalFrictionForce - brakeForce;

% Equations of motion
positionDot = velocity;
velocityDot = force/mass;
